simulink model "model_3_extended"  (R2021b)
settings: Solver=VariableStepAuto  StartTime=0.0  StopTime=10.0  RelTol=1e-3
undefined symbols (not defined in the file): A, B, C, K, L
settings Model: Creator=den  LastModifiedBy=den

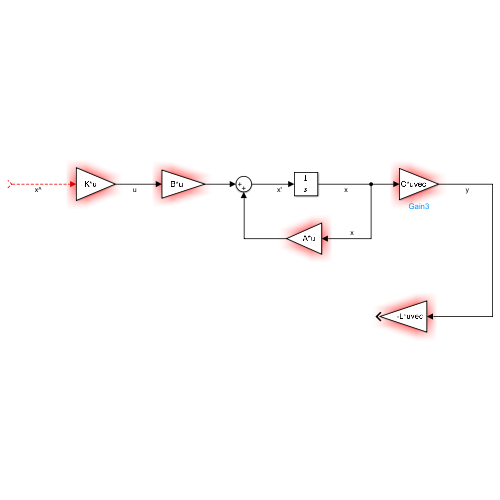
[thumbnail: Simulink's stored preview of the top-level diagram]
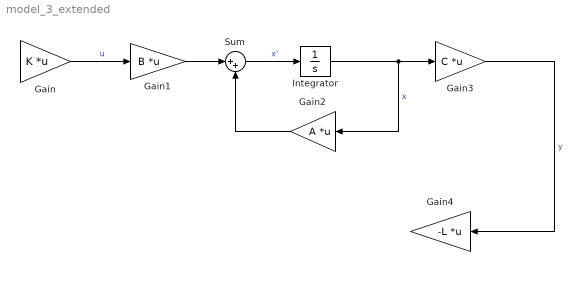
== system model_3_extended ==
  Gain : Gain  Gain=K  Multiplication=Matrix(K*u)
  Gain1 : Gain  Gain=B  Multiplication=Matrix(K*u)
  Gain2 : Gain  Gain=A  Multiplication=Matrix(K*u)
  Gain3 : Gain  Gain=C  Multiplication=Matrix(K*u) (u vector)
  Gain4 : Gain  Gain=-L  Multiplication=Matrix(K*u) (u vector)
  Integrator : Integrator
  Sum : Sum  Inputs=|++
  wires:
  Gain/1 -> Gain1/1  "u"
  ? -> Gain/1  "x^"
  Gain1/1 -> Sum/1
  Gain2/1 -> Sum/2
  Integrator/1 -> Gain3/1, Gain2/1  "x"
  Sum/1 -> Integrator/1  "x'"
  Gain3/1 -> Gain4/1  "y"
